simulink model "Nuas_JIA_Simulink_No4"  (R2023b)
settings: Solver=VariableStepAuto  StartTime=0.0  StopTime=20  RelTol=1e-3
values from neighbouring files (symbols this model uses):
  G_den4 = [M,B,K]    [NUAS_JIA_NO_4 _AND_5.m]
  G_num4 = [1]    [NUAS_JIA_NO_4 _AND_5.m]
settings Model: Creator=justine  LastModifiedBy=justine

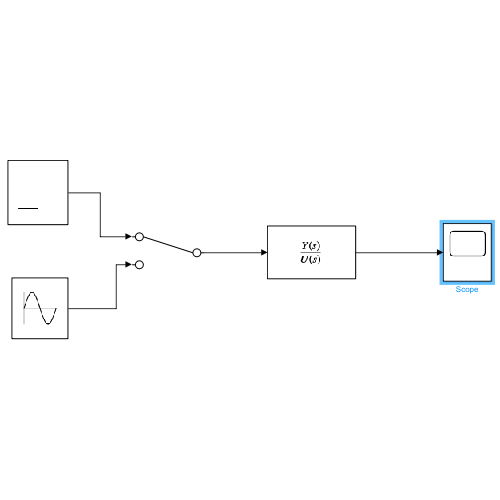
[thumbnail: Simulink's stored preview of the top-level diagram]
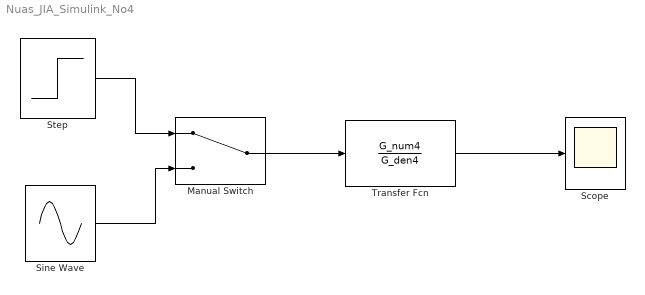
== system Nuas_JIA_Simulink_No4 ==
  Manual Switch : ManualSwitch
  Scope : Scope
  Sine Wave : Sin  SampleTime=0
  Step : Step  SampleTime=0
  Transfer Fcn : TransferFcn  Numerator=G_num4  Denominator=G_den4
  wires:
  Step/1 -> Manual Switch/1
  Sine Wave/1 -> Manual Switch/2
  Manual Switch/1 -> Transfer Fcn/1
  Transfer Fcn/1 -> Scope/1
